simulink model "ex1_8"  (Simulink 8.1)
settings: Solver=ode45  StartTime=0.0  StopTime=600  RelTol=1e-3
values from neighbouring files (symbols this model uses):
  a0 = 1    [task2.m]
  a0_c = 1    [task2.m]
  a1 = a10+delta_a1    (= 3.4)    [task2.m]
  a1_c = 0    [task2.m]
  a2 = a20+delta_a2    (= 4)    [task2.m]
  a2_c = we(i)^2    [task2.m]
  b0_c = 1    [task2.m]
  b1_c = 1    [task2.m]
  b2_c = 1    [task2.m]
  w = linspace(0,5,size(windSpectrum,1))    [task2.m]
settings Model: Creator=Nelson  LastModifiedBy=Nelson
settings DataIOCC: SignalLoggingSaveFormat=Dataset
settings OptimizationCC: ExpressionDepthLimit=128
settings DebuggingCC: FcnCallInpInsideContextMsg=EnableAllAsError
settings GRTTargetCC: CombineOutputUpdateFcns=on  GRTInterface=off

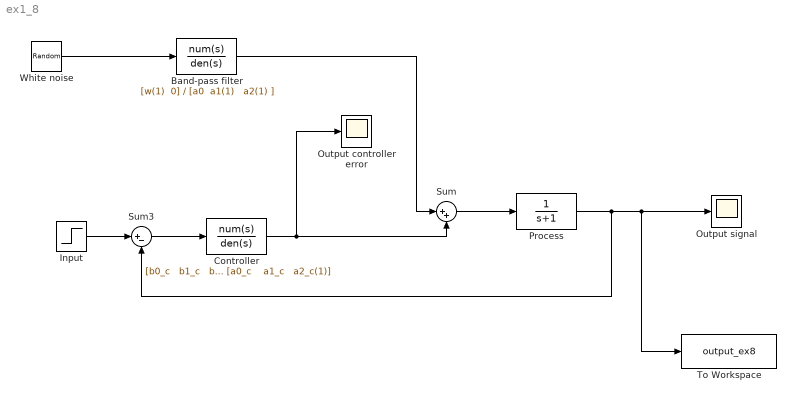
== system ex1_8 ==
  Band-pass filter : TransferFcn  Numerator="[w(1)  0]"  Denominator="[a0  a1(1)   a2(1) ]"
  Controller : TransferFcn  Numerator="[b0_c   b1_c   b2_c]"  Denominator="[a0_c    a1_c   a2_c(1)]"  AbsoluteTolerance=0.1
  Input : Step  Time=0  VectorParams1D=off
  Output controller error : Scope
  "Output signal " : Scope
  Process : TransferFcn  Denominator=[1 1]
  Sum : Sum  Inputs=|++
  Sum3 : Sum  Inputs=|+-
  To Workspace : ToWorkspace  VariableName=output_ex8  SampleTime=-1  SaveFormat=Structure
  White noise : RandomNumber  VectorParams1D=off
  wires:
  White noise/1 -> Band-pass filter/1
  Band-pass filter/1 -> Sum/1
  Input/1 -> Sum3/1
  Sum3/1 -> Controller/1
  Process/1 -> Sum3/2, "Output signal "/1, To Workspace/1
  Sum/1 -> Process/1
  Controller/1 -> Sum/2, Output controller error/1
